simulink model "missile_trim_model"  (R2022b)
settings: Solver=VariableStepAuto  StartTime=0.0  StopTime=10.0  RelTol=1e-3
InitFcn:
  | % clc, clear, close all
  | UAV_Data
  | Sim_Parameters
values from neighbouring files (symbols this model uses):
  Alt_Trim = 0    [Missile_Trim_Solution.mat]    (also in Trim_Main_missile.m = 4000; Trim_Solution_missile1.mat; Trim_Solution_missile2.mat; Trim_Solution_missile3.mat)
  D = 0.150    (= 0.15)    [UAV_Data.m]    (also in UAV_Data.mat)
  G_Turn = Turn_dot_Trim * Speed_Trim / UNIT_GRAV    [Trim_Main_missile.m]
  Gamma_Trim = 0.0 * UNIT_DEG2RAD    [Trim_Main_missile.m]
  I_TENSOR = [ I_xx,  0.0,  0.0 ... (first row only)    [UAV_Data.m]    (also in UAV_Data.mat = [0.084375  0  0; 0  6.5869975  0; 0  0  6.5869975])
  Init_Cnstr1 = 0.0    (= 0)    [Trim_Main_missile.m]
  Init_Cnstr2 = 0.0    (= 0)    [Trim_Main_missile.m]
  Init_Cnstr3 = 0.0    (= 0)    [Trim_Main_missile.m]
  Init_Euler = [ 0, 0.0, 0.0 ] *  UNIT_DEG2RAD    [Sim_Parameters.m]    (also in main_Assigment3.m = [ 0.0, 0.0, 0.0 ]')
  Init_Rate = [ 0, 0.0, 0.0 ] * UNIT_DEG2RAD    [Sim_Parameters.m]    (also in main_Assigment3.m = [ 0.0, 0.0, 0.0 ]')
  Init_Vel = [ 238.0, 0.0, 0.0 ]    [Sim_Parameters.m]    (also in main_Assigment3.m = [ 238, 0, 0]')
  Mass = 30.0    (= 30)    [UAV_Data.m]    (also in UAV_Data.mat)
  S = dat.S    [Assigment3_work.m]    (also in Missile_EoM.m; UAV_Data.m = 0.0176714586764; UAV_Data.mat = 0.0176714586764; verify_coeff.m)
  Speed_Trim = 102.088237307    [Missile_Trim_Solution.mat]    (also in Trim_Main_missile.m = 227.1878; Trim_Solution_missile1.mat = 102.0804; Trim_Solution_missile2.mat = 136.1072; Trim_Solution_missile3.mat = 204.1608)
  Theta_dot_Trim = 0.0 * UNIT_DEG2RAD    [Trim_Main_missile.m]
  Turn_dot_Trim = 0.0 * UNIT_DEG2RAD    [Trim_Main_missile.m]
  UNIT_GRAV = 9.81    [Sim_Parameters.m]
libraries: aerolibasang x2, shared6dofsys x2, aerolibtransform2 x1, sharedtransform x1, sharedutil x1, aerolibatmos2 x1
settings Model: Creator=Komsun  LastModifiedBy=Komsun

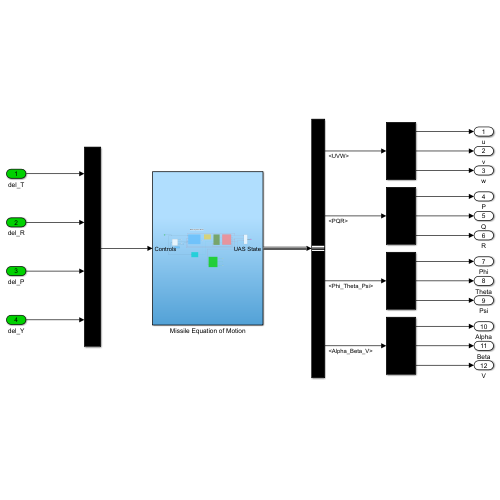
[thumbnail: Simulink's stored preview of the top-level diagram]
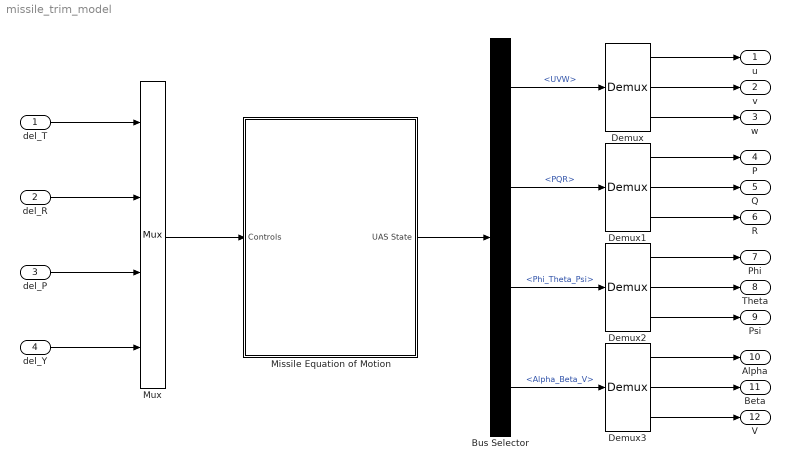
== system missile_trim_model ==
  del_T : Inport
  del_R : Inport  Port=2
  del_P : Inport  Port=3
  del_Y : Inport  Port=4
  Bus Selector : BusSelector  OutputSignals=UVW,PQR,Phi_Theta_Psi,Alpha_Beta_V
  Demux{,1..3} (4 alike) : Demux  Outputs=3
  Missile Equation of Motion : Subsystem
  Mux : Mux
  u : Outport
  v : Outport  Port=2
  w : Outport  Port=3
  P : Outport  Port=4
  Q : Outport  Port=5
  R : Outport  Port=6
  Phi : Outport  Port=7
  Theta : Outport  Port=8
  Psi : Outport  Port=9
  Alpha : Outport  Port=10
  Beta : Outport  Port=11
  V : Outport  Port=12
  wires:
  Demux1/1 -> P/1
  Demux2/3 -> Psi/1
  del_T/1 -> Mux/1
  Demux3/2 -> Beta/1
  Demux1/3 -> R/1
  Demux/1 -> u/1
  Demux/3 -> w/1
  Demux/2 -> v/1
  Demux3/3 -> V/1
  Mux/1 -> Missile Equation of Motion/1(Controls)
  Demux2/1 -> Phi/1
  del_P/1 -> Mux/3
  del_R/1 -> Mux/2
  Demux1/2 -> Q/1
  del_Y/1 -> Mux/4
  Demux2/2 -> Theta/1
  Missile Equation of Motion/1(UAS State) -> Bus Selector/1
  Bus Selector/1 -> Demux/1  "<UVW>"
  Bus Selector/2 -> Demux1/1  "<PQR>"
  Bus Selector/3 -> Demux2/1  "<Phi_Theta_Psi>"
  Bus Selector/4 -> Demux3/1  "<Alpha_Beta_V>"
  Demux3/1 -> Alpha/1

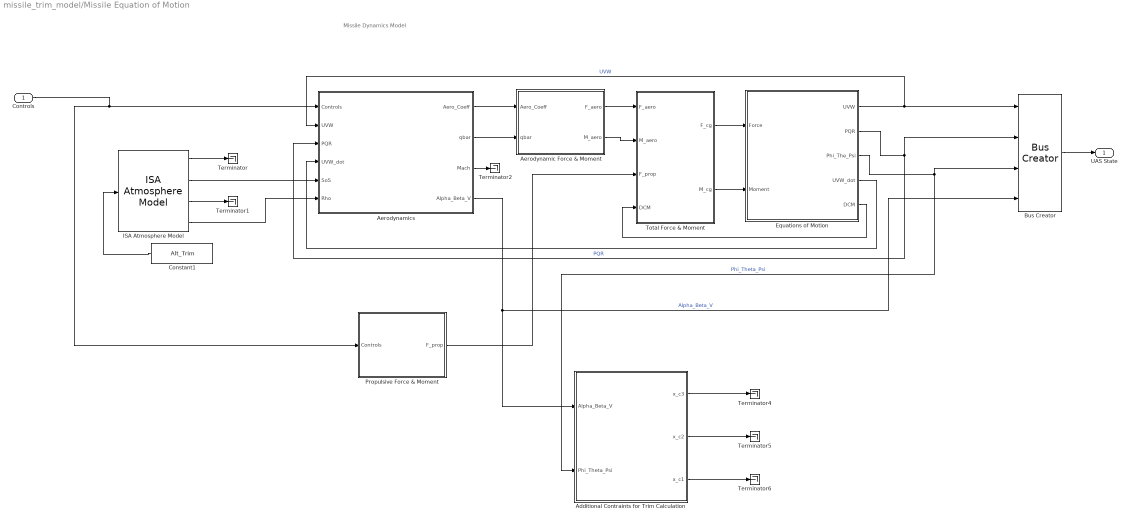
== system missile_trim_model/Missile Equation of Motion ==
  note: Missile Dynamics Model
  Controls : Inport
  Additional Contraints for Trim Calculation : Subsystem
  Aerodynamic Force & Moment : Subsystem
  Aerodynamics : Subsystem
  Bus Creator : BusCreator  Inputs=4
  Constant1 : Constant  Value=Alt_Trim
  Equations of Motion : Subsystem
  ISA Atmosphere Model : aerolibatmos2/ISA Atmosphere Model  custom=off  g=9.80665  gamma=1.4  R=287.0531  L=0.0065  h_trop=11000  h_strat=20000  rho0=1.225  P0=101325  T0=288.15  h0=0
  Propulsive Force & Moment : Subsystem
  Terminator{,1..2,4..6} (6 alike) : Terminator
  Total Force & Moment : Subsystem
  UAS State : Outport
  wires:
  Aerodynamics/4(Alpha_Beta_V) -> Bus Creator/4, Additional Contraints for Trim Calculation/1(Alpha_Beta_V)  "Alpha_Beta_V"
  Propulsive Force & Moment/1(F_prop) -> Total Force & Moment/3(F_prop)
  Constant1/1 -> ISA Atmosphere Model/1
  ISA Atmosphere Model/2 -> Aerodynamics/5(SoS)
  Aerodynamics/1(Aero_Coeff) -> Aerodynamic Force & Moment/1(Aero_Coeff)
  Aerodynamic Force & Moment/1(F_aero) -> Total Force & Moment/1(F_aero)
  ISA Atmosphere Model/1 -> Terminator/1
  ISA Atmosphere Model/3 -> Terminator1/1
  Controls/1 -> Propulsive Force & Moment/1(Controls), Aerodynamics/1(Controls)
  Aerodynamic Force & Moment/2(M_aero) -> Total Force & Moment/2(M_aero)
  Aerodynamics/3(Mach) -> Terminator2/1
  Aerodynamics/2(qbar) -> Aerodynamic Force & Moment/2(qbar)
  Total Force & Moment/1(F_cg) -> Equations of Motion/1(Force)
  Total Force & Moment/2(M_cg) -> Equations of Motion/2(Moment)
  ISA Atmosphere Model/4 -> Aerodynamics/6(Rho)
  Bus Creator/1 -> UAS State/1
  Additional Contraints for Trim Calculation/1(x_c3) -> Terminator4/1
  Additional Contraints for Trim Calculation/3(x_c1) -> Terminator6/1
  Additional Contraints for Trim Calculation/2(x_c2) -> Terminator5/1
  Equations of Motion/1(UVW) -> Bus Creator/1, Aerodynamics/2(UVW)  "UVW"
  Equations of Motion/2(PQR) -> Bus Creator/2, Aerodynamics/3(PQR)  "PQR"
  Equations of Motion/3(Phi_The_Psi) -> Bus Creator/3, Additional Contraints for Trim Calculation/2(Phi_Theta_Psi)  "Phi_Theta_Psi"
  Equations of Motion/4(UVW_dot) -> Aerodynamics/4("UVW_dot ")
  Equations of Motion/5(DCM) -> Total Force & Moment/4(DCM)

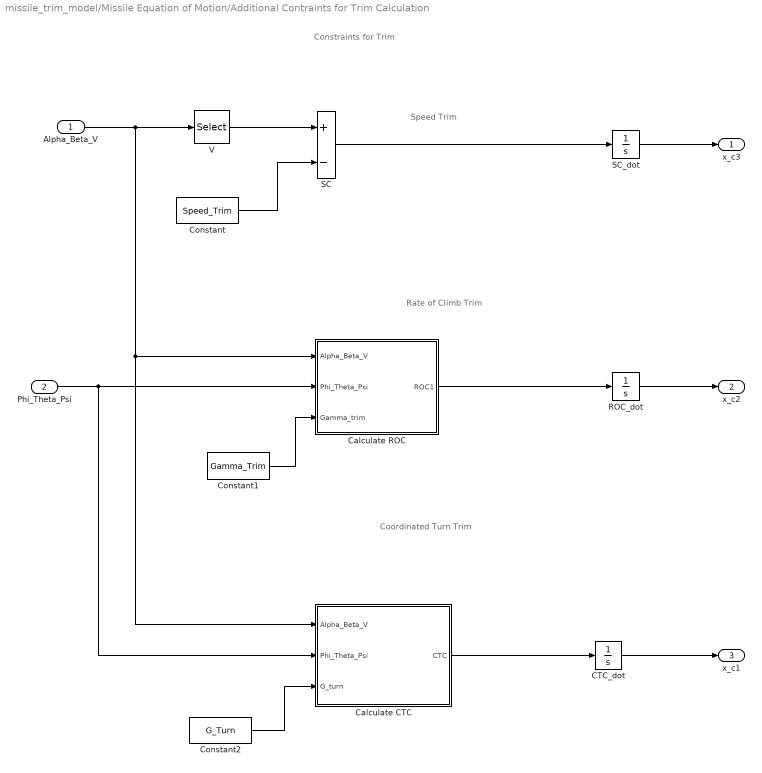
== system missile_trim_model/Missile Equation of Motion/Additional Contraints for Trim Calculation ==
  note: Speed Trim
  note: Constraints for Trim
  note: Coordinated Turn Trim
  note: Rate of Climb Trim
  Alpha_Beta_V : Inport  PortDimensions=3
  Phi_Theta_Psi : Inport  Port=2  PortDimensions=3
  CTC_dot : Integrator  InitialCondition=Init_Cnstr3
  Calculate CTC : Subsystem
  Calculate ROC : Subsystem
  Constant : Constant  Value=Speed_Trim
  Constant1 : Constant  Value=Gamma_Trim
  Constant2 : Constant  Value=G_Turn
  ROC_dot : Integrator  InitialCondition=Init_Cnstr2
  SC : Sum  Inputs=+-
  SC_dot : Integrator  InitialCondition=Init_Cnstr1
  V : Selector  InputPortWidth=3  IndexOptions=Index vector (dialog)  Indices=[3]  OutputSizes=1
  x_c3 : Outport
  x_c2 : Outport  Port=2
  x_c1 : Outport  Port=3
  wires:
  SC_dot/1 -> x_c3/1
  ROC_dot/1 -> x_c2/1
  CTC_dot/1 -> x_c1/1
  Alpha_Beta_V/1 -> Calculate CTC/1(Alpha_Beta_V), Calculate ROC/1(Alpha_Beta_V), V/1
  V/1 -> SC/1
  Constant/1 -> SC/2
  SC/1 -> SC_dot/1
  Constant2/1 -> Calculate CTC/3(G_turn)
  Phi_Theta_Psi/1 -> Calculate CTC/2(Phi_Theta_Psi), Calculate ROC/2(Phi_Theta_Psi)
  Constant1/1 -> Calculate ROC/3(Gamma_trim)
  Calculate ROC/1(ROC1) -> ROC_dot/1
  Calculate CTC/1(CTC) -> CTC_dot/1

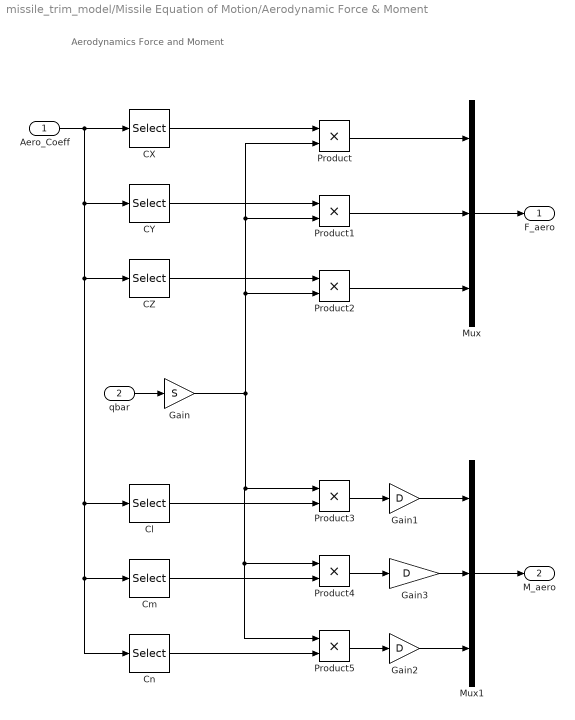
== system missile_trim_model/Missile Equation of Motion/Aerodynamic Force & Moment ==
  note: Aerodynamics Force and Moment
  Aero_Coeff : Inport
  qbar : Inport  Port=2
  CX : Selector  InputPortWidth=6  IndexOptions=Index vector (dialog)  Indices=[1]  OutputSizes=1
  CY : Selector  InputPortWidth=6  IndexOptions=Index vector (dialog)  Indices=[2]  OutputSizes=1
  CZ : Selector  InputPortWidth=6  IndexOptions=Index vector (dialog)  Indices=[3]  OutputSizes=1
  Cl : Selector  InputPortWidth=6  IndexOptions=Index vector (dialog)  Indices=[4]  OutputSizes=1
  Cm : Selector  InputPortWidth=6  IndexOptions=Index vector (dialog)  Indices=[5]  OutputSizes=1
  Cn : Selector  InputPortWidth=6  IndexOptions=Index vector (dialog)  Indices=[6]  OutputSizes=1
  Gain : Gain  Gain=S
  Gain1 : Gain  Gain=D
  Gain2 : Gain  Gain=D
  Gain3 : Gain  Gain=D
  Mux : Mux  Inputs=3
  Mux1 : Mux  Inputs=3
  Product{,1..5} (6 alike) : Product
  F_aero : Outport
  M_aero : Outport  Port=2
  wires:
  Aero_Coeff/1 -> Cl/1, Cn/1, Cm/1, CZ/1, CY/1, CX/1
  qbar/1 -> Gain/1
  CX/1 -> Product/1
  Gain/1 -> Product5/1, Product4/1, Product3/1, Product2/2, Product1/2, Product/2
  CY/1 -> Product1/1
  CZ/1 -> Product2/1
  Product/1 -> Mux/1
  Product1/1 -> Mux/2
  Product2/1 -> Mux/3
  Mux/1 -> F_aero/1
  Cl/1 -> Product3/2
  Cm/1 -> Product4/2
  Cn/1 -> Product5/2
  Product3/1 -> Gain1/1
  Product4/1 -> Gain3/1
  Product5/1 -> Gain2/1
  Mux1/1 -> M_aero/1
  Gain1/1 -> Mux1/1
  Gain2/1 -> Mux1/3
  Gain3/1 -> Mux1/2

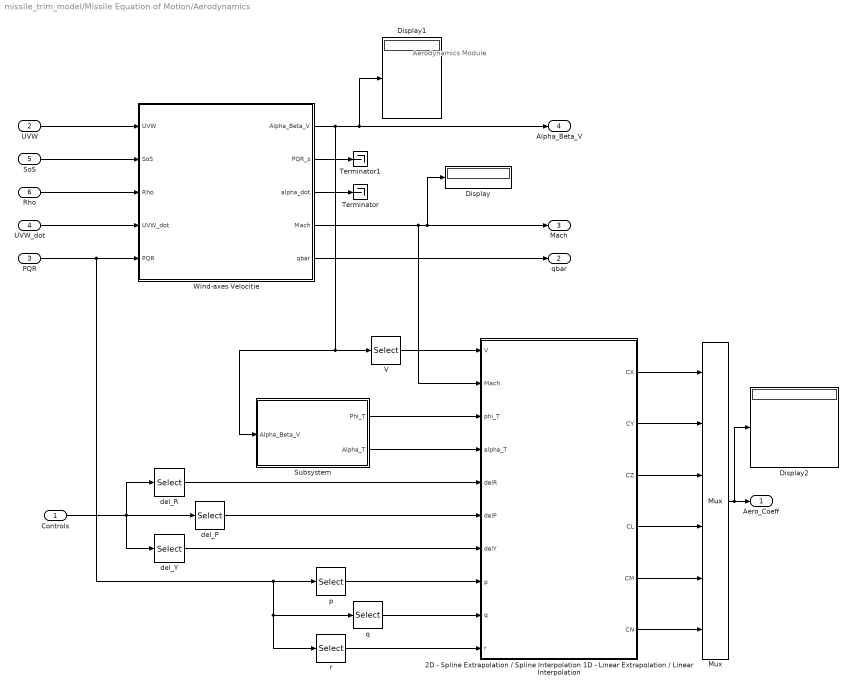
== system missile_trim_model/Missile Equation of Motion/Aerodynamics ==
  note: Aerodynamics Module
  Controls : Inport
  UVW : Inport  Port=2
  PQR : Inport  Port=3
  "UVW_dot " : Inport  Port=4
  SoS : Inport  Port=5
  Rho : Inport  Port=6
  2D - Spline Extrapolation / Spline Interpolation 1D - Linear Extrapolation / Linear Interpolation : MATLAB Function  TreatAsAtomicUnit=on
  Display : Display
  Display1 : Display
  Display2 : Display
  Mux : Mux  Inputs=6
  Subsystem : Subsystem
  Terminator : Terminator
  Terminator1 : Terminator
  V : Selector  InputPortWidth=3  IndexOptions=Index vector (dialog)  Indices=[3]  OutputSizes=1
  Wind-axes Velocitie : Subsystem
  del_P : Selector  InputPortWidth=4  IndexOptions=Index vector (dialog)  Indices=[3]  OutputSizes=1
  del_R : Selector  InputPortWidth=4  IndexOptions=Index vector (dialog)  Indices=[2]  OutputSizes=1
  del_Y : Selector  InputPortWidth=4  IndexOptions=Index vector (dialog)  Indices=[4]  OutputSizes=1
  p : Selector  InputPortWidth=3  IndexOptions=Index vector (dialog)  Indices=[1]  OutputSizes=1
  q : Selector  InputPortWidth=3  IndexOptions=Index vector (dialog)  Indices=[2]  OutputSizes=1
  r : Selector  InputPortWidth=3  IndexOptions=Index vector (dialog)  Indices=[3]  OutputSizes=1
  Aero_Coeff : Outport
  qbar : Outport  Port=2
  Mach : Outport  Port=3
  Alpha_Beta_V : Outport  Port=4
  wires:
  Wind-axes Velocitie/1(Alpha_Beta_V) -> Subsystem/1(Alpha_Beta_V), V/1, Display1/1, Alpha_Beta_V/1
  UVW/1 -> Wind-axes Velocitie/1(UVW)
  Mux/1 -> Display2/1, Aero_Coeff/1
  Wind-axes Velocitie/4(Mach) -> 2D - Spline Extrapolation / Spline Interpolation 1D - Linear Extrapolation / Linear Interpolation/2(Mach), Mach/1, Display/1
  Wind-axes Velocitie/5(qbar) -> qbar/1
  SoS/1 -> Wind-axes Velocitie/2(SoS)
  Rho/1 -> Wind-axes Velocitie/3(Rho)
  "UVW_dot "/1 -> Wind-axes Velocitie/4(UVW_dot)
  PQR/1 -> r/1, q/1, p/1, Wind-axes Velocitie/5(PQR)
  Wind-axes Velocitie/3(alpha_dot) -> Terminator/1
  Wind-axes Velocitie/2(PQR_s) -> Terminator1/1
  Subsystem/2(Alpha_T) -> 2D - Spline Extrapolation / Spline Interpolation 1D - Linear Extrapolation / Linear Interpolation/4(alpha_T)
  V/1 -> 2D - Spline Extrapolation / Spline Interpolation 1D - Linear Extrapolation / Linear Interpolation/1(V)
  Subsystem/1(Phi_T) -> 2D - Spline Extrapolation / Spline Interpolation 1D - Linear Extrapolation / Linear Interpolation/3(phi_T)
  Controls/1 -> del_Y/1, del_R/1, del_P/1
  del_Y/1 -> 2D - Spline Extrapolation / Spline Interpolation 1D - Linear Extrapolation / Linear Interpolation/7(delY)
  p/1 -> 2D - Spline Extrapolation / Spline Interpolation 1D - Linear Extrapolation / Linear Interpolation/8(p)
  q/1 -> 2D - Spline Extrapolation / Spline Interpolation 1D - Linear Extrapolation / Linear Interpolation/9(q)
  r/1 -> 2D - Spline Extrapolation / Spline Interpolation 1D - Linear Extrapolation / Linear Interpolation/10(r)
  2D - Spline Extrapolation / Spline Interpolation 1D - Linear Extrapolation / Linear Interpolation/1(CX) -> Mux/1
  2D - Spline Extrapolation / Spline Interpolation 1D - Linear Extrapolation / Linear Interpolation/2(CY) -> Mux/2
  2D - Spline Extrapolation / Spline Interpolation 1D - Linear Extrapolation / Linear Interpolation/3(CZ) -> Mux/3
  2D - Spline Extrapolation / Spline Interpolation 1D - Linear Extrapolation / Linear Interpolation/4(CL) -> Mux/4
  2D - Spline Extrapolation / Spline Interpolation 1D - Linear Extrapolation / Linear Interpolation/5(CM) -> Mux/5
  2D - Spline Extrapolation / Spline Interpolation 1D - Linear Extrapolation / Linear Interpolation/6(CN) -> Mux/6
  del_P/1 -> 2D - Spline Extrapolation / Spline Interpolation 1D - Linear Extrapolation / Linear Interpolation/6(delP)
  del_R/1 -> 2D - Spline Extrapolation / Spline Interpolation 1D - Linear Extrapolation / Linear Interpolation/5(delR)

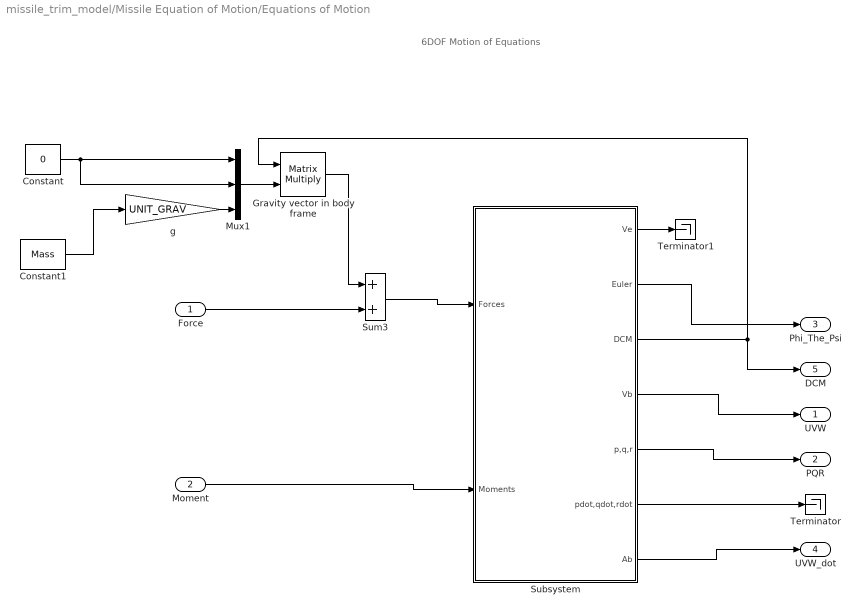
== system missile_trim_model/Missile Equation of Motion/Equations of Motion ==
  note: 6DOF Motion of Equations
  Force : Inport  PortDimensions=3
  Moment : Inport  Port=2  PortDimensions=3
  Constant : Constant  Value=0
  Constant1 : Constant  Value=Mass
  "Gravity vector in body frame " : Product  Multiplication=Matrix(*)  InputSameDT=on  SaturateOnIntegerOverflow=on  OutDataTypeStr=Inherit: Same as first input
  Mux1 : Mux  Inputs=3
  Subsystem : Subsystem
  Sum3 : Sum  InputSameDT=on  SaturateOnIntegerOverflow=on  OutDataTypeStr=Inherit: Same as first input
  Terminator : Terminator
  Terminator1 : Terminator
  g : Gain  Gain=UNIT_GRAV
  UVW : Outport
  PQR : Outport  Port=2
  Phi_The_Psi : Outport  Port=3
  UVW_dot : Outport  Port=4
  DCM : Outport  Port=5
  wires:
  Sum3/1 -> Subsystem/1(Forces)
  g/1 -> Mux1/3
  "Gravity vector in body frame "/1 -> Sum3/1
  Constant/1 -> Mux1/2, Mux1/1
  Mux1/1 -> "Gravity vector in body frame "/2
  Force/1 -> Sum3/2
  Moment/1 -> Subsystem/2(Moments)
  Constant1/1 -> g/1
  Subsystem/2(Euler) -> Phi_The_Psi/1
  Subsystem/3(DCM) -> DCM/1, "Gravity vector in body frame "/1
  Subsystem/4(Vb) -> UVW/1
  Subsystem/5(p,q,r) -> PQR/1
  Subsystem/6(pdot,qdot,rdot) -> Terminator/1
  Subsystem/7(Ab) -> UVW_dot/1
  Subsystem/1(Ve) -> Terminator1/1

== system missile_trim_model/Missile Equation of Motion/Propulsive Force & Moment ==
  note: Propulsive Force and Moment
  Controls : Inport
  Constant : Constant  Value=0
  Mux : Mux  Inputs=3
  Thrust : Selector  InputPortWidth=4  IndexOptions=Index vector (dialog)  Indices=[1]  OutputSizes=1
  F_prop : Outport
  wires:
  Constant/1 -> Mux/3, Mux/2
  Controls/1 -> Thrust/1
  Thrust/1 -> Mux/1
  Mux/1 -> F_prop/1

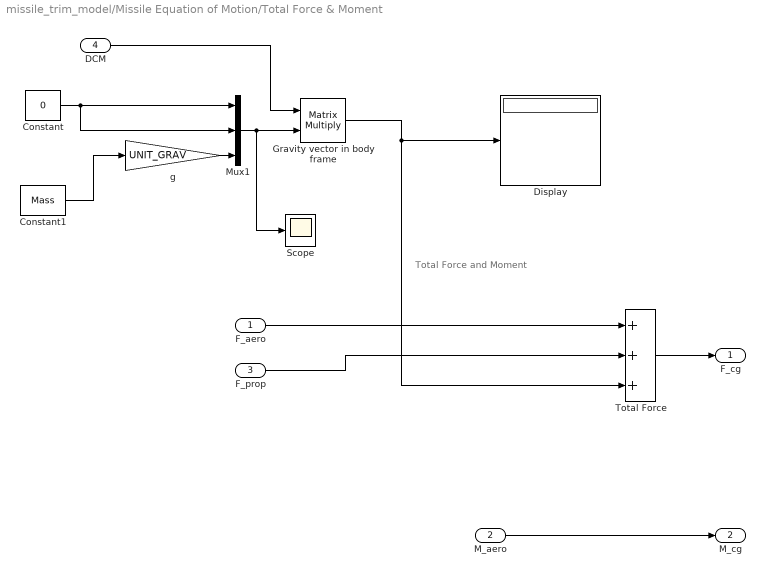
== system missile_trim_model/Missile Equation of Motion/Total Force & Moment ==
  note: Total Force and Moment
  F_aero : Inport  PortDimensions=3
  M_aero : Inport  Port=2  PortDimensions=3
  F_prop : Inport  Port=3  PortDimensions=3
  DCM : Inport  Port=4
  Constant : Constant  Value=0
  Constant1 : Constant  Value=Mass
  Display : Display
  "Gravity vector in body frame " : Product  Multiplication=Matrix(*)  InputSameDT=on  SaturateOnIntegerOverflow=on  OutDataTypeStr=Inherit: Same as first input
  Mux1 : Mux  Inputs=3
  Scope : Scope
  Total Force : Sum  Inputs=+++  InputSameDT=on  SaturateOnIntegerOverflow=on  OutDataTypeStr=Inherit: Same as first input
  g : Gain  Gain=UNIT_GRAV
  F_cg : Outport
  M_cg : Outport  Port=2
  wires:
  Total Force/1 -> F_cg/1
  F_aero/1 -> Total Force/1
  F_prop/1 -> Total Force/2
  M_aero/1 -> M_cg/1
  Mux1/1 -> Scope/1, "Gravity vector in body frame "/2
  "Gravity vector in body frame "/1 -> Total Force/3, Display/1
  Constant1/1 -> g/1
  Constant/1 -> Mux1/2, Mux1/1
  g/1 -> Mux1/3
  DCM/1 -> "Gravity vector in body frame "/1

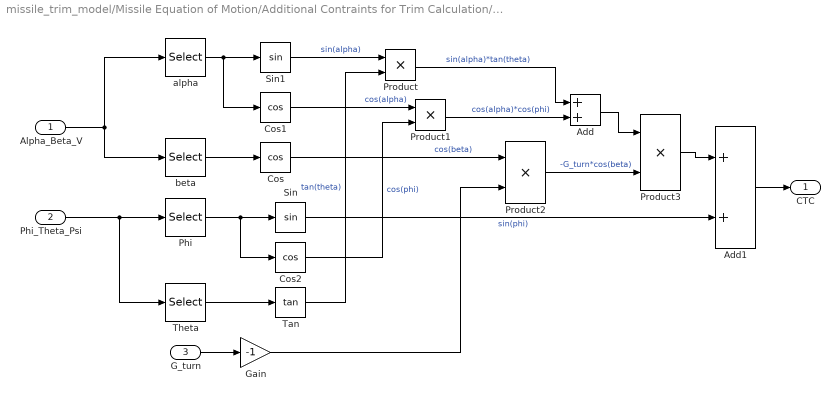
== system missile_trim_model/Missile Equation of Motion/Additional Contraints for Trim Calculation/Calculate CTC ==
  Alpha_Beta_V : Inport
  Phi_Theta_Psi : Inport  Port=2
  G_turn : Inport  Port=3
  Add : Sum
  Add1 : Sum
  Cos : Trigonometry  Operator=cos
  Cos1 : Trigonometry  Operator=cos
  Cos2 : Trigonometry  Operator=cos
  Gain : Gain  Gain=-1
  Phi : Selector  InputPortWidth=3  IndexOptions=Index vector (dialog)  Indices=[1]  OutputSizes=1
  Product{,1..3} (4 alike) : Product
  Sin : Trigonometry
  Sin1 : Trigonometry
  Tan : Trigonometry  Operator=tan
  Theta : Selector  InputPortWidth=3  IndexOptions=Index vector (dialog)  Indices=[2]  OutputSizes=1
  alpha : Selector  InputPortWidth=3  IndexOptions=Index vector (dialog)  Indices=[1]  OutputSizes=1
  beta : Selector  InputPortWidth=3  IndexOptions=Index vector (dialog)  Indices=[2]  OutputSizes=1
  CTC : Outport
  wires:
  Alpha_Beta_V/1 -> alpha/1, beta/1
  Phi_Theta_Psi/1 -> Theta/1, Phi/1
  Phi/1 -> Cos2/1, Sin/1
  Sin/1 -> Add1/2  "sin(phi)"
  G_turn/1 -> Gain/1
  beta/1 -> Cos/1
  alpha/1 -> Cos1/1, Sin1/1
  Theta/1 -> Tan/1
  Tan/1 -> Product/2  "tan(theta)"
  Sin1/1 -> Product/1  "sin(alpha)"
  Cos/1 -> Product2/1  "cos(beta)"
  Product/1 -> Add/1  "sin(alpha)*tan(theta)"
  Cos1/1 -> Product1/1  "cos(alpha)"
  Cos2/1 -> Product1/2  "cos(phi)"
  Product1/1 -> Add/2  "cos(alpha)*cos(phi)"
  Gain/1 -> Product2/2
  Product2/1 -> Product3/2  "-G_turn*cos(beta)"
  Add/1 -> Product3/1
  Product3/1 -> Add1/1
  Add1/1 -> CTC/1

== system missile_trim_model/Missile Equation of Motion/Additional Contraints for Trim Calculation/Calculate ROC ==
  Alpha_Beta_V : Inport
  Phi_Theta_Psi : Inport  Port=2
  Gamma_trim : Inport  Port=3
  ROC : Subsystem
  Theta : Selector  InputPortWidth=3  IndexOptions=Index vector (dialog)  Indices=[2]  OutputSizes=1
  calculate a : Subsystem
  calculate b : Subsystem
  ROC1 : Outport
  wires:
  Gamma_trim/1 -> ROC/4(Gamma_trim)
  Phi_Theta_Psi/1 -> calculate b/2(Phi_Theta_Psi), Theta/1
  calculate a/1(a) -> ROC/1(a)
  Alpha_Beta_V/1 -> calculate a/1(Alpha_Beta_V), calculate b/1(Alpha_Beta_V)
  ROC/1(ROC) -> ROC1/1
  Theta/1 -> ROC/3(Theta)
  calculate b/1(b) -> ROC/2(b)

== system missile_trim_model/Missile Equation of Motion/Aerodynamics/Subsystem ==
  Alpha_Beta_V : Inport
  Acos : Trigonometry  Operator=acos
  Atan2 : Trigonometry  Operator=atan2
  Beta : Selector  InputPortWidth=3  IndexOptions=Index vector (dialog)  Indices=[2]  OutputSizes=1
  Cos1 : Trigonometry  Operator=cos
  Cos2 : Trigonometry  Operator=cos
  Product : Product
  Sin : Trigonometry
  Tan : Trigonometry  Operator=tan
  alpha : Selector  InputPortWidth=3  IndexOptions=Index vector (dialog)  Indices=[1]  OutputSizes=1
  Phi_T : Outport
  Alpha_T : Outport  Port=2
  wires:
  Alpha_Beta_V/1 -> alpha/1, Beta/1
  Beta/1 -> Tan/1, Cos2/1
  Tan/1 -> Atan2/1
  Sin/1 -> Atan2/2
  Atan2/1 -> Phi_T/1
  alpha/1 -> Cos1/1, Sin/1
  Cos1/1 -> Product/1
  Cos2/1 -> Product/2
  Product/1 -> Acos/1
  Acos/1 -> Alpha_T/1

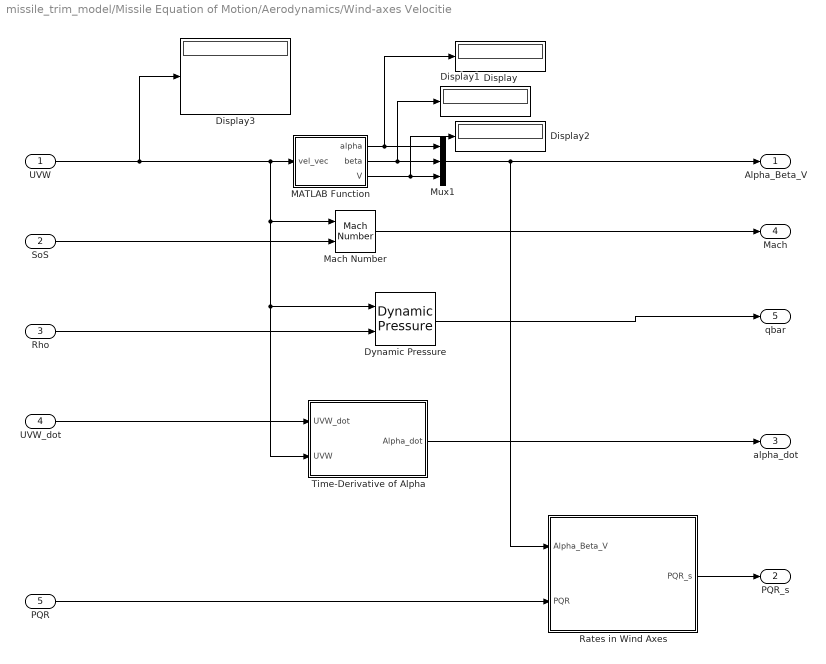
== system missile_trim_model/Missile Equation of Motion/Aerodynamics/Wind-axes Velocitie ==
  UVW : Inport
  SoS : Inport  Port=2
  Rho : Inport  Port=3
  UVW_dot : Inport  Port=4
  PQR : Inport  Port=5
  Display{,1..3} (4 alike) : Display
  Dynamic Pressure : aerolibasang/Dynamic Pressure
  MATLAB Function : MATLAB Function  TreatAsAtomicUnit=on
  Mach Number : aerolibasang/Mach Number
  Mux1 : Mux  Inputs=3
  Rates in Wind Axes : Subsystem
  Time-Derivative of Alpha : Subsystem
  Alpha_Beta_V : Outport
  PQR_s : Outport  Port=2
  alpha_dot : Outport  Port=3
  Mach : Outport  Port=4
  qbar : Outport  Port=5
  wires:
  UVW_dot/1 -> Time-Derivative of Alpha/1(UVW_dot)
  Time-Derivative of Alpha/1(Alpha_dot) -> alpha_dot/1
  Dynamic Pressure/1 -> qbar/1
  Rho/1 -> Dynamic Pressure/2
  SoS/1 -> Mach Number/2
  Mach Number/1 -> Mach/1
  Mux1/1 -> Rates in Wind Axes/1(Alpha_Beta_V), Alpha_Beta_V/1
  UVW/1 -> Display3/1, Mach Number/1, Time-Derivative of Alpha/2(UVW), Dynamic Pressure/1, MATLAB Function/1(vel_vec)
  MATLAB Function/1(alpha) -> Mux1/1, Display/1
  MATLAB Function/2(beta) -> Mux1/2, Display1/1
  MATLAB Function/3(V) -> Display2/1, Mux1/3
  Rates in Wind Axes/1(PQR_s) -> PQR_s/1
  PQR/1 -> Rates in Wind Axes/2(PQR)

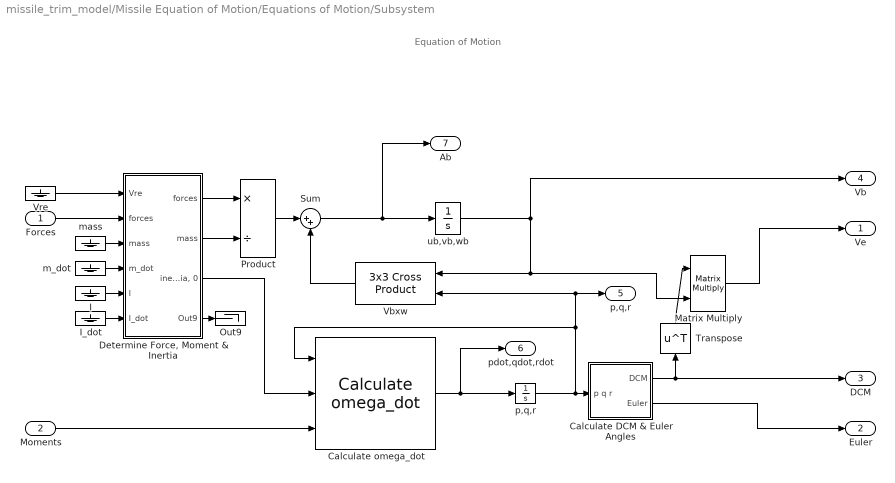
== system missile_trim_model/Missile Equation of Motion/Equations of Motion/Subsystem ==
  note: Equation of Motion
  Forces : Inport  PortDimensions=3
  Moments : Inport  Port=2  PortDimensions=3
  Calculate DCM & Euler Angles : Subsystem
  Calculate omega_dot : shared6dofsys/Calculate omega_dot  aMode=aMode
  "Determine Force, Moment & Inertia" : Subsystem
  I : Ground
  I_dot : Ground
  Matrix Multiply : Product  Multiplication=Matrix(*)
  Out9 : Terminator
  Product : Product  Inputs=*/  SaturateOnIntegerOverflow=on  OutDataTypeStr=Inherit: Same as first input
  Sum : Sum  Inputs=|++  SaturateOnIntegerOverflow=on
  Transpose : Math  Operator=transpose  SignedPower=on
  Vbxw : sharedutil/3x3 Cross Product  aMode=aMode
      settings: LibrarySourceBlock=aerolibutil/3x3 Cross Product
  Vre : Ground
  m_dot : Ground
  mass : Ground
  "p,q,r " : Integrator  InitialCondition=Init_Rate
  ub,vb,wb : Integrator  InitialCondition=Init_Vel
  Ve : Outport
  Euler : Outport  Port=2
  DCM : Outport  Port=3
  Vb : Outport  Port=4
  p,q,r : Outport  Port=5
  pdot,qdot,rdot : Outport  Port=6
  Ab : Outport  Port=7
  wires:
  Matrix Multiply/1 -> Ve/1
  ub,vb,wb/1 -> Vb/1, Matrix Multiply/2, Vbxw/1
  Vre/1 -> "Determine Force, Moment & Inertia"/1(Vre)
  "Determine Force, Moment & Inertia"/1("forces ") -> Product/1
  I_dot/1 -> "Determine Force, Moment & Inertia"/6(I_dot)
  I/1 -> "Determine Force, Moment & Inertia"/5(I)
  Calculate omega_dot/1 -> "p,q,r "/1, pdot,qdot,rdot/1
  "Determine Force, Moment & Inertia"/4(Out9) -> Out9/1
  m_dot/1 -> "Determine Force, Moment & Inertia"/4(m_dot)
  mass/1 -> "Determine Force, Moment & Inertia"/3("mass ")
  Transpose/1 -> Matrix Multiply/1
  Calculate DCM & Euler Angles/1(DCM) -> Transpose/1, DCM/1
  Product/1 -> Sum/1
  Forces/1 -> "Determine Force, Moment & Inertia"/2(forces)
  Moments/1 -> Calculate omega_dot/3
  "p,q,r "/1 -> Calculate DCM & Euler Angles/1("p q r "), Vbxw/2, p,q,r/1, Calculate omega_dot/1
  Vbxw/1 -> Sum/2
  Calculate DCM & Euler Angles/2(Euler) -> Euler/1
  "Determine Force, Moment & Inertia"/2(mass) -> Product/2
  "Determine Force, Moment & Inertia"/3("inertia, 0") -> Calculate omega_dot/2
  Sum/1 -> Ab/1, ub,vb,wb/1

== system missile_trim_model/Missile Equation of Motion/Additional Contraints for Trim Calculation/Calculate ROC/ROC ==
  a : Inport
  b : Inport  Port=2
  Theta : Inport  Port=3
  Gamma_trim : Inport  Port=4
  Add : Sum  Inputs=+++
  Cos : Trigonometry  Operator=cos
  Gain : Gain  Gain=-1
  Product : Product
  Product1 : Product
  Sin : Trigonometry
  Sin1 : Trigonometry
  ROC : Outport
  wires:
  Gamma_trim/1 -> Sin/1
  Theta/1 -> Cos/1, Sin1/1
  b/1 -> Product/1
  Cos/1 -> Product/2
  Product/1 -> Add/1  "b*cos(theta)"
  Sin1/1 -> Product1/1
  a/1 -> Gain/1
  Product1/1 -> Add/2  "-a*sin(theta)"
  Gain/1 -> Product1/2
  Sin/1 -> Add/3  "sin(Gamma_trim)"
  Add/1 -> ROC/1

== system missile_trim_model/Missile Equation of Motion/Additional Contraints for Trim Calculation/Calculate ROC/calculate a ==
  Alpha_Beta_V : Inport
  Cos : Trigonometry  Operator=cos
  Cos1 : Trigonometry  Operator=cos
  Product : Product
  alpha : Selector  InputPortWidth=3  IndexOptions=Index vector (dialog)  Indices=[1]  OutputSizes=1
  beta : Selector  InputPortWidth=3  IndexOptions=Index vector (dialog)  Indices=[2]  OutputSizes=1
  a : Outport
  wires:
  alpha/1 -> Cos/1
  beta/1 -> Cos1/1
  Cos/1 -> Product/1
  Cos1/1 -> Product/2
  Alpha_Beta_V/1 -> beta/1, alpha/1
  Product/1 -> a/1

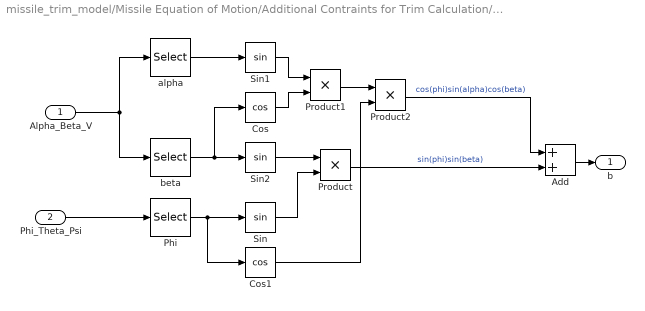
== system missile_trim_model/Missile Equation of Motion/Additional Contraints for Trim Calculation/Calculate ROC/calculate b ==
  Alpha_Beta_V : Inport
  Phi_Theta_Psi : Inport  Port=2
  Add : Sum
  Cos : Trigonometry  Operator=cos
  Cos1 : Trigonometry  Operator=cos
  Phi : Selector  InputPortWidth=3  IndexOptions=Index vector (dialog)  Indices=[1]  OutputSizes=1
  Product : Product
  Product1 : Product
  Product2 : Product
  Sin : Trigonometry
  Sin1 : Trigonometry
  Sin2 : Trigonometry
  alpha : Selector  InputPortWidth=3  IndexOptions=Index vector (dialog)  Indices=[1]  OutputSizes=1
  beta : Selector  InputPortWidth=3  IndexOptions=Index vector (dialog)  Indices=[2]  OutputSizes=1
  b : Outport
  wires:
  Alpha_Beta_V/1 -> beta/1, alpha/1
  Phi_Theta_Psi/1 -> Phi/1
  Phi/1 -> Cos1/1, Sin/1
  alpha/1 -> Sin1/1
  beta/1 -> Cos/1, Sin2/1
  Sin2/1 -> Product/1
  Sin/1 -> Product/2
  Product/1 -> Add/2  "sin(phi)sin(beta)"
  Sin1/1 -> Product1/1
  Cos/1 -> Product1/2
  Product1/1 -> Product2/1
  Cos1/1 -> Product2/2
  Product2/1 -> Add/1  "cos(phi)sin(alpha)cos(beta)"
  Add/1 -> b/1

== system missile_trim_model/Missile Equation of Motion/Aerodynamics/Wind-axes Velocitie/Rates in Wind Axes ==
  note: Rates in Wind Axes
  Alpha_Beta_V : Inport
  PQR : Inport  Port=2
  Alpha : Selector  InputPortWidth=3  IndexOptions=Index vector (dialog)  Indices=[1]  OutputSizes=1
  Beta_Ref : Constant  Value=0
  Direction Cosine Matrix Body to Wind : aerolibtransform2/Direction Cosine Matrix Body to Wind
  Mux : Mux  Inputs=2
  transform to body axes : Product  Inputs=**  Multiplication=Matrix(*)  InputSameDT=on  SaturateOnIntegerOverflow=on  OutDataTypeStr=Inherit: Same as first input
  PQR_s : Outport
  wires:
  Alpha_Beta_V/1 -> Alpha/1
  Alpha/1 -> Mux/1
  Direction Cosine Matrix Body to Wind/1 -> transform to body axes/1  "cB_W"
  PQR/1 -> transform to body axes/2
  transform to body axes/1 -> PQR_s/1
  Mux/1 -> Direction Cosine Matrix Body to Wind/1
  Beta_Ref/1 -> Mux/2

== system missile_trim_model/Missile Equation of Motion/Aerodynamics/Wind-axes Velocitie/Time-Derivative of Alpha ==
  note: Time Derivative of Alpha
  UVW_dot : Inport
  UVW : Inport  Port=2
  Add : Sum  Inputs=-+
  Add1 : Sum
  Demux2 : Demux  Outputs=3
  Demux3 : Demux  Outputs=3
  Divide : Product  Inputs=*/
  Math Function2 : Math  Operator=square  SignedPower=on
  Math Function3 : Math  Operator=square  SignedPower=on
  Product3 : Product
  Product4 : Product
  Terminator2 : Terminator
  Terminator3 : Terminator
  Alpha_dot : Outport
  wires:
  UVW_dot/1 -> Demux2/1
  Demux2/2 -> Terminator2/1
  Demux2/1 -> Product3/1
  UVW/1 -> Demux3/1
  Demux3/2 -> Terminator3/1
  Demux3/3 -> Math Function3/1, Product3/2
  Demux2/3 -> Product4/1
  Demux3/1 -> Math Function2/1, Product4/2
  Product4/1 -> Add/2
  Product3/1 -> Add/1
  Add/1 -> Divide/1
  Math Function2/1 -> Add1/1
  Math Function3/1 -> Add1/2
  Add1/1 -> Divide/2
  Divide/1 -> Alpha_dot/1

== system missile_trim_model/Missile Equation of Motion/Equations of Motion/Subsystem/Calculate DCM & Euler Angles ==
  "p q r " : Inport
  Constant : Constant  Value=Theta_dot_Trim
  Constant1 : Constant  Value=Turn_dot_Trim
  Demux : Demux  Outputs=3
  Mux : Mux  Inputs=3
  Rotation Angles to Direction Cosine Matrix : sharedtransform/Rotation Angles to Direction Cosine Matrix  rotationOrder=ZYX  aMode=aMode
  Selector : Selector  InputPortWidth=3  IndexOptions=Index vector (dialog)  Indices=[3 2 1]  OutputSizes=1
  Sum : Sum  Inputs=|+-
  Sum1 : Sum  Inputs=|+-
  phi theta psi : Integrator  InitialCondition=Init_Euler
  phidot thetadot psidot : shared6dofsys/DCM & Euler Angles (Euler)/phidot thetadot psidot  SystemSampleTime=-1  VariantActivationTime=update diagram  Latency=0  AutoFrameSizeCalculation=off
  DCM : Outport
  Euler : Outport  Port=2
  wires:
  Selector/1 -> Rotation Angles to Direction Cosine Matrix/1
  phi theta psi/1 -> phidot thetadot psidot/2, Selector/1, Euler/1
  "p q r "/1 -> phidot thetadot psidot/1
  Rotation Angles to Direction Cosine Matrix/1 -> DCM/1
  phidot thetadot psidot/1 -> Demux/1
  Mux/1 -> phi theta psi/1
  Demux/1 -> Mux/1
  Demux/2 -> Sum/1
  Constant/1 -> Sum/2
  Sum/1 -> Mux/2
  Sum1/1 -> Mux/3
  Demux/3 -> Sum1/1
  Constant1/1 -> Sum1/2

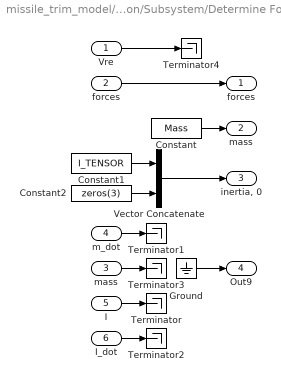
== system missile_trim_model/Missile Equation of Motion/Equations of Motion/Subsystem/Determine Force, Moment & Inertia ==
  Vre : Inport
  forces : Inport  Port=2
  "mass " : Inport  Port=3
  m_dot : Inport  Port=4  OutDataTypeStr=double
  I : Inport  Port=5  OutDataTypeStr=double
  I_dot : Inport  Port=6  OutDataTypeStr=double
  Constant : Constant  Value=Mass  OutDataTypeStr=Inherit: Inherit via back propagation
  Constant1 : Constant  Value=I_TENSOR  OutDataTypeStr=Inherit: Inherit via back propagation
  Constant2 : Constant  Value=zeros(3)
  Ground : Ground
  Terminator{,1..4} (5 alike) : Terminator
  Vector Concatenate : Concatenate  Mode=Multidimensional array
  "forces " : Outport
  mass : Outport  Port=2
  "inertia, 0" : Outport  Port=3
  Out9 : Outport  Port=4
  wires:
  Vector Concatenate/1 -> "inertia, 0"/1
  Constant2/1 -> Vector Concatenate/2
  Constant1/1 -> Vector Concatenate/1
  Vre/1 -> Terminator4/1
  forces/1 -> "forces "/1
  "mass "/1 -> Terminator3/1
  I_dot/1 -> Terminator2/1
  m_dot/1 -> Terminator1/1
  I/1 -> Terminator/1
  Ground/1 -> Out9/1
  Constant/1 -> mass/1

== matlab function missile_trim_model/Missile Equation of Motion/Aerodynamics/Wind-axes Velocitie/MATLAB Function ==
  data: vel_vec input; alpha output; beta output; V output
function [alpha, beta, V] = calc_abv(vel_vec)

u = vel_vec(1);
v = vel_vec(2);
w = vel_vec(3);

V = norm([u v w]);          % [m/s] UAV total Speed
% V = sqrt(u^2 + v^2 + w^2);
alpha = atan2(w,u);          % [rad] angle of attack
% alpha = atan(w/u);          % [rad] angle of attack
beta  = asin(v/V);          % [rad] sideslip angles

end

== matlab function missile_trim_model/Missile Equation of Motion/Aerodynamics/2D - Spline Extrapolation // Spline Interpolation 1D - Linear Extrapolation // Linear Interpolation ==
  data: V input; Mach input; CX output; phi_T input; alpha_T input; delR input; delP input; delY input; CY output; CZ output; CL output; CM output; CN output; p input; q input; r input
function [CX, CY, CZ, CL, CM, CN] = AeroCoef(V, Mach,phi_T, alpha_T, delR, delP, delY, p, q, r)

dat = load('UAV_Data.mat');
dat.Tbl_ALPHAT = dat.Tbl_ALPHAT;    % convert to rad
% alpha_T = alpha_T *180/pi;            % convert to degree

del_eff = (abs(delP) + abs(delY))/2;


B2A = rot1(-phi_T);                            % Body-to-Aeroballistics

delARPY = B2A *[delR; delP; delY];
delR_A = delARPY(1);
delP_A = delARPY(2);
delY_A = delARPY(3);

pqrA = B2A * [p; q; r];
pA = pqrA(1);
qA = pqrA(2);
rA = pqrA(3);

method = 'linear'; % 'spline', 'nearest'
method2 = 'spline';

CX_a = interp1(dat.Tbl_MACH, dat.Tbl_CX_0, Mach, method,'extrap') + interp1(dat.Tbl_MACH, dat.Tbl_CX_ALPHAT, Mach, method,'extrap')*alpha_T...
     + interp1(dat.Tbl_MACH, dat.Tbl_CX_DEL_EFF, Mach, method,'extrap')*(del_eff)^2;

CY_a = interp2(dat.Tbl_ALPHAT, dat.Tbl_MACH, dat.Tbl_CY_PHIT, alpha_T*180/pi, Mach, method2)*sin(4*phi_T)...
     + interp1(dat.Tbl_MACH, dat.Tbl_CY_DEL_Y, Mach, method,'extrap')*delY_A;

CZ_a = interp2(dat.Tbl_ALPHAT, dat.Tbl_MACH, dat.Tbl_CZ_0, alpha_T*180/pi, Mach, method2)...
     + interp2(dat.Tbl_ALPHAT, dat.Tbl_MACH, dat.Tbl_CZ_PHIT, alpha_T*180/pi, Mach, method2)*(sin(2*phi_T))^2 ...
     + interp1(dat.Tbl_MACH, dat.Tbl_CZ_DEL_P, Mach, method,'extrap')*delP_A;

CL_a = interp1(dat.Tbl_MACH, dat.Tbl_CL_ALPHAT, Mach, method,'extrap')*(alpha_T^2)*sin(4*phi_T) ...
     + interp1(dat.Tbl_MACH, dat.Tbl_CL_P, Mach, method,'extrap')*(dat.D/(2*V))*pA ...
     + interp1(dat.Tbl_MACH, dat.Tbl_CL_DEL_R, Mach, method,'extrap')*delR_A;

CM_a = interp2(dat.Tbl_ALPHAT, dat.Tbl_MACH, dat.Tbl_CM_0, alpha_T*180/pi, Mach, method2) ...
     + interp2(dat.Tbl_ALPHAT, dat.Tbl_MACH, dat.Tbl_CM_PHIT, alpha_T*180/pi, Mach, method2)*(sin(2*phi_T))^2 ...
     + interp1(dat.Tbl_MACH, dat.Tbl_CM_Q, Mach, method,'extrap')*(dat.D/(2*V))*qA ...
     + interp1(dat.Tbl_MACH, dat.Tbl_CM_DEL_P, Mach, method,'extrap')*delP_A ...
     - CZ_a*(dat.XCG - dat.XREF)/dat.D;

CN_a = interp2(dat.Tbl_ALPHAT, dat.Tbl_MACH, dat.Tbl_CN_PHIT, alpha_T*180/pi, Mach, method2)*sin(4*phi_T)...
     + interp1(dat.Tbl_MACH, dat.Tbl_CN_R, Mach, method,'extrap')*(dat.D/(2*V))*rA ...
     + interp1(dat.Tbl_MACH, dat.Tbl_CN_DEL_Y, Mach, method,'extrap')*delY_A ...
     + CY_a*(dat.XCG - dat.XREF)/dat.D;

%% Aerodynamics Coefficients in body coordinate


CXYZ = B2A.' * [CX_a; CY_a; CZ_a];
CX = CXYZ(1);
CY = CXYZ(2);
CZ = CXYZ(3);

CLMN = B2A.' * [CL_a; CM_a; CN_a];
CL = CLMN(1);
CM = CLMN(2);
CN = CLMN(3);

function out = rot1(x)
    out = [1 0 0; 0 cos(x) sin(x); 0 -sin(x) cos(x)];
end

end
